simulink model "ACDCMG_woPV"  (R2022a)
settings: Solver=FixedStepAuto  StartTime=0.0  StopTime=0.2  FixedStep=Ts  MaxStep=1e-2  RelTol=1e-3
InitFcn:
  | Set_parameters_R2018
values from neighbouring files (symbols this model uses):
  D_invs = 0.05    [Set_parameters_R2018.m]
  dis11 = 3    [Set_parameters_R2018.m]
  dis14 = 2    [Set_parameters_R2018.m]
  dis2 = 0.2    [Set_parameters_R2018.m]
  dis3 = 0.15    [Set_parameters_R2018.m]
  dis4 = 0.4    [Set_parameters_R2018.m]
  dis5 = 0.4    [Set_parameters_R2018.m]
  dis6 = 0.4    [Set_parameters_R2018.m]
  dis8 = 2    [Set_parameters_R2018.m]
  Fnom = 60    [Set_parameters_R2018.m]
  H_invs = 6    [Set_parameters_R2018.m]
  max_min = 1    [Set_parameters_R2018.m]
  P_Load_3 = S_Load_3* PF_Load_3    (= 25500)    [Set_parameters_R2018.m]
  P_nom_inv = 3e3    (= 3000)    [Set_parameters_R2018.m]
  Pnom_T1 = 1.5e6    (= 1500000)    [Set_parameters_R2018.m]
  Pnom_T2 = 1.5e6    (= 1500000)    [Set_parameters_R2018.m]
  Pnom_T3 = 4e6    (= 4000000)    [Set_parameters_R2018.m]
  Ql_Load_3 = S_Load_3 * sin(acos(PF_Load_3))    [Set_parameters_R2018.m]
  R_Load_9 = (Vnom_prim * 1.35)^2 / P_Load_9    (= 1084.6153125)    [Set_parameters_R2018.m]
  R_Load_DC = Vnom_DC^2/ P_Load_DC    (= 45)    [Set_parameters_R2018.m]
  Rl = 0.394    [Set_parameters_R2018.m]
  Rls = 0.198    [Set_parameters_R2018.m]
  Ts = Ts_Power    (= 6.94444444444e-06)    [Set_parameters_R2018.m]
  Ts_Control = 6*Ts_Power    (= 4.16666666667e-05)    [Set_parameters_R2018.m]
  Ts_Power = 1/(24*Fnom)/100    (= 6.94444444444e-06)    [Set_parameters_R2018.m]
  V1_LL_T3 = 69e3    (= 69000)    [Set_parameters_R2018.m]
  Vnom_DC = 300    [Set_parameters_R2018.m]
  Vnom_Diesel = 2.4e3    (= 2400)    [Set_parameters_R2018.m]
  Vnom_prim = 13.8e3    (= 13800)    [Set_parameters_R2018.m]
  Vnom_sec = 220    [Set_parameters_R2018.m]
  Vnom_ter_AC_DC = 150    [Set_parameters_R2018.m]
  Xl = 0.1168    [Set_parameters_R2018.m]
  Xls = 0.1089    [Set_parameters_R2018.m]
undefined symbols (not defined in the file or in its folder): D1, Delta, DiscIntNeverNeededParam, ee_sli_rtmsupport, fn, gcbh, Ion, Lithium, S, sigbuilder_block, VnInv
libraries: powerlib_extras x55, spsCurrentMeasurementLib x53, powerlib_meascontrol x42, spsSeriesRLCBranchLib x32, spsVoltageMeasurementLib x31, spsRMSLib x29, spsThreePhaseVIMeasurementLib x24, simulink x21, spsThreePhaseSeriesRLCBranchLib x19, spsPower3phInstantaneousLib x15, spsPowerLib x12, spsGroundLib x11
(part 9 of 9)

== system ACDCMG_woPV/Grid Bi-directional Converter 1.2 300 (DC) // 150 V (AC) P_nom 3kW3/Control of Inverter/V//F/Subsystem ==
  note: w
  e : Inport
  io : Inport  Port=2
  i : Inport  Port=3
  fcmd : Inport  Port=4
  Constant1 : Constant  Value=2*pi
  Demux : Demux  Outputs=3
  Demux1 : Demux  Outputs=3
  Demux2 : Demux  Outputs=3
  Discrete Virtual PLL : powerlib_extras/Discrete  Control Blocks/Discrete Virtual PLL  Commented=on  Freq=50  Phase=0  Ts=Ts_Control
      settings: SourceProductBaseCode=PS
  Gain1 : Gain  Gain=2*pi
  Integrator : Integrator
  Math Function : Math  Operator=mod  SignedPower=on
  Scope : Scope
  Scope3 : Scope
  Terminator1 : Terminator
  Terminator2 : Terminator
  Terminator3 : Terminator
  Terminator4 : Terminator  Commented=on
  abc to dq0 : powerlib_meascontrol/Transformations/abc to dq0  Alignment=90 degrees behind phase A axis
  abc to dq1 : powerlib_meascontrol/Transformations/abc to dq0  Alignment=90 degrees behind phase A axis
  abc to dq2 : powerlib_meascontrol/Transformations/abc to dq0  Alignment=90 degrees behind phase A axis
  abc_to_dq0 Transformation2 : powerlib_extras/Measurements/abc_to_dq0 Transformation  Commented=on
      settings: SourceProductBaseCode=PS
  pack6 Scope1 : Scope  NumInputPorts=2
  ed : Outport
  eq : Outport  Port=2
  iod : Outport  Port=3
  ioq : Outport  Port=4
  id : Outport  Port=5
  iq : Outport  Port=6
  w : Outport  Port=7
  "wt " : Outport  Port=8
  wires:
  e/1 -> abc to dq0/1
  i/1 -> abc to dq1/1
  fcmd/1 -> Gain1/1
  Math Function/1 -> Scope3/1, abc to dq1/2, abc to dq2/2, abc to dq0/2, "wt "/1
  abc to dq0/1 -> Demux/1
  Demux1/1 -> id/1
  Demux1/2 -> iq/1
  Demux1/3 -> Terminator3/1
  Demux/1 -> ed/1
  Demux/2 -> eq/1
  Demux/3 -> Terminator1/1
  abc to dq1/1 -> Demux1/1
  Constant1/1 -> Math Function/2
  Integrator/1 -> Math Function/1
  io/1 -> abc to dq2/1
  abc to dq2/1 -> Demux2/1
  Demux2/3 -> Terminator2/1
  Gain1/1 -> Scope/1, w/1, Integrator/1
  Discrete Virtual PLL/2 -> Terminator4/1
  Demux2/1 -> pack6 Scope1/1, iod/1
  Demux2/2 -> pack6 Scope1/2, ioq/1

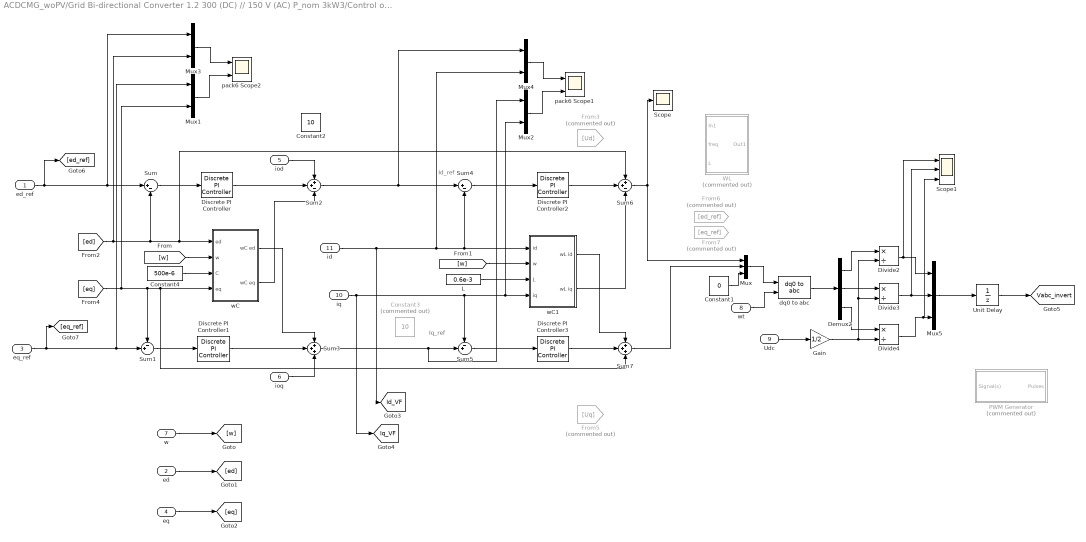
== system ACDCMG_woPV/Grid Bi-directional Converter 1.2 300 (DC) // 150 V (AC) P_nom 3kW3/Control of Inverter/V//F/UIcontrol ==
  note: Id_ref
  note: Iq_ref
  ed_ref : Inport
  ed : Inport  Port=2
  eq_ref : Inport  Port=3
  eq : Inport  Port=4
  iod : Inport  Port=5
  ioq : Inport  Port=6
  w : Inport  Port=7
  "wt " : Inport  Port=8
  Udc : Inport  Port=9
  iq : Inport  Port=10
  id : Inport  Port=11
  Constant1 : Constant  Value=0
  Constant2 : Constant  Value=10
  Constant3 : Constant  Commented=on  Value=10
  Constant4 : Constant  Value=500e-6
  Demux2 : Demux  Outputs=3
  Discrete PI Controller : powerlib_extras/Discrete  Control Blocks/Discrete PI Controller  Kp=5  Ki=50  Par_Limits=[1e6 -1e6]  Init=0  Ts=Ts_Control
  Discrete PI Controller1 : powerlib_extras/Discrete  Control Blocks/Discrete PI Controller  Kp=5  Ki=50  Par_Limits=[1e6 -1e6]  Init=0  Ts=Ts_Control
  Discrete PI Controller2 : powerlib_extras/Discrete  Control Blocks/Discrete PI Controller  Kp=25  Ki=1800  Par_Limits=[1e6 -1e6]  Init=0  Ts=Ts_Control
  Discrete PI Controller3 : powerlib_extras/Discrete  Control Blocks/Discrete PI Controller  Kp=25  Ki=1800  Par_Limits=[1e6 -1e6]  Init=0  Ts=Ts_Control
  Divide2 : Product  Inputs=*/
  Divide3 : Product  Inputs=*/
  Divide4 : Product  Inputs=*/
  From3 : From  Commented=on  GotoTag=Ud
  From5 : From  Commented=on  GotoTag=Uq
  From6 : From  Commented=on  GotoTag=ed_ref
  From7 : From  Commented=on  GotoTag=eq_ref
  Gain : Gain  Gain=1/2
  L : Constant  Value=0.6e-3
  Mux : Mux  Inputs=3
  Mux{1..4} (4 alike) : Mux  Inputs=2
  Mux5 : Mux  Inputs=3
  PWM Generator : Subsystem  Commented=on  AncestorBlock="powerlib_extras/Control  Blocks/PWM Generator"  DialogController=POWERSYS.PowerSysDialog  mask(PWM Generator){GeneratorMode=3-arm  bridge (6 pulses), Fc=10000, Internal=off, mIndex=0.4, Freq=50, Phase=0}
      mask prompts: GeneratorMode "Generator Mode"; Fc "Carrier frequency (Hz):"; Internal "Internal generation of modulating signal(s)"; mIndex "Modulation index  (0<m<1) :"; Freq "Frequency of output voltage (Hz)"; Phase "Phase of output voltage (degrees)"
      mask help:
      | This block generates pulses for carrier-based PWM (Pulse Width Modulation), self-commutated IGBTs,GTOs or FETs bridges.
      |
      | Depending on the number of bridge arms selected in the "Generator Mode" parameter, the block can be used either for single-phase or three-phase PWM control.
      mask init: same as ACDCMG_woPV/Grid Bi-directional Converter 1.2 300 (DC) // 150 V (AC) P_nom 3kW/Control of Inverter/V//F/UIcontrol/PWM Generator
      mask Help: web(psbhelp)
      mask TypeOptions GeneratorMode: 1-arm  bridge (2 pulses) | 2-arm  bridge (4 pulses) | 3-arm  bridge (6 pulses) | Double 3-arm  bridges (12 pulses)
      mask Callback Internal: p3=get_param(gcb,'Internal');if strcmp(p3,'on');visible={'on','on','on','on','on','on'};else;visible={'on','on','on','off','off','off'};end;set_param(gcb,'MaskVisibilities',visible)
  Scope : Scope
  Scope1 : Scope  NumInputPorts=3
  Sum : Sum  Inputs=|+-
  Sum1 : Sum  Inputs=-+|
  Sum2 : Sum  Inputs=++-
  Sum3 : Sum  Inputs=+++
  Sum4 : Sum  Inputs=|+-
  Sum5 : Sum  Inputs=-+|
  Sum6 : Sum  Inputs=++-
  Sum7 : Sum  Inputs=+++
  Unit Delay : UnitDelay  SampleTime=-1  HasFrameUpgradeWarning=on
  WL : Subsystem  Commented=on
  dq0 to abc : powerlib_meascontrol/Transformations/dq0 to abc  Alignment=90 degrees behind phase A axis
  pack6 Scope1 : Scope  NumInputPorts=2
  pack6 Scope2 : Scope  NumInputPorts=2
  wC : Subsystem
  wC1 : Subsystem
  tag scope: Id_VF=global, Iq_VF=global, Vabc_invert=global
  wires:
  ed_ref/1 -> [ed_ref], Mux3/1, Sum/1
  Sum/1 -> Discrete PI Controller/1
  Mux/1 -> dq0 to abc/1
  "wt "/1 -> dq0 to abc/2
  Mux5/1 -> Unit Delay/1
  Demux2/1 -> Divide2/1
  Demux2/2 -> Divide3/1
  Gain/1 -> Divide3/2, Divide2/2, Divide4/2
  Divide4/1 -> Scope1/3, Mux5/3
  Divide2/1 -> Mux5/1, Scope1/1
  Demux2/3 -> Divide4/1
  Divide3/1 -> Scope1/2, Mux5/2
  dq0 to abc/1 -> Demux2/1
  Udc/1 -> Gain/1
  Constant4/1 -> wC/3(C)
  [w] -> wC/2(w)
  [eq] -> Mux1/2, Sum7/3, wC/4(eq), Sum1/1
  Sum1/1 -> Discrete PI Controller1/1
  eq_ref/1 -> [eq_ref], Mux1/1, Sum1/2
  L/1 -> wC1/3(L)
  Sum5/1 -> Discrete PI Controller3/1
  Sum4/1 -> Discrete PI Controller2/1
  Discrete PI Controller3/1 -> Sum7/2
  Discrete PI Controller2/1 -> Sum6/2
  w/1 -> [w]
  [w] -> wC1/2(w)
  ed/1 -> [ed]
  eq/1 -> [eq]
  Sum6/1 -> Mux/1, Scope/1
  Constant1/1 -> Mux/3
  Mux4/1 -> pack6 Scope1/1
  Mux2/1 -> pack6 Scope1/2
  iq/1 -> [Iq_VF], Sum5/1, wC1/4(iq), Mux2/2
  Discrete PI Controller/1 -> Sum2/2
  Discrete PI Controller1/1 -> Sum3/2
  id/1 -> [Id_VF], Mux4/2, wC1/1(id), Sum4/2
  Mux3/1 -> pack6 Scope2/1
  Mux1/1 -> pack6 Scope2/2
  wC/1(wC ed) -> Sum3/1
  ioq/1 -> Sum3/3
  iod/1 -> Sum2/1
  wC/2(wC eq) -> Sum2/3
  wC1/1(wL id) -> Sum7/1
  wC1/2(wL iq) -> Sum6/3
  [ed] -> Sum6/1, wC/1(ed), Sum/2, Mux3/2
  Sum2/1 -> Mux4/1, Sum4/1
  Sum3/1 -> Mux2/1, Sum5/2
  Unit Delay/1 -> [Vabc_invert]
  Sum7/1 -> Mux/2

== system ACDCMG_woPV/Inverter 300 (DC) // 150 V (AC) P_nom 3kW4/Control of Inverter/Subsystem2/Subsystem1 ==
  note: Iq* = 2/3*( P*Vq - Q*Vd ) / ( Vd^2 + Vq^2 )
  note: Reference computation:
  note: Id* = 2/3* ( P*Vd + Q*Vq ) / ( Vd^2 + Vq^2 )
  P_ref : Inport  PortDimensions=1
  Q_ref : Inport  Port=2  PortDimensions=1
  Vd : Inport  Port=3  PortDimensions=1
  Vq : Inport  Port=4  PortDimensions=1
  Constant1 : Constant  Commented=on  Value=0
  Demux3 : Demux  Outputs=2
      settings: DisplayOption=none
  Fcn3 : Fcn  Expr=u(1)*u(1)+u(2)*u(2)
  Gain : Gain  Gain=2/3
  Mux1 : Mux  Inputs=2
  Mux3 : Mux  Inputs=2
  Product{2..5} (4 alike) : Product  InputSameDT=on  SaturateOnIntegerOverflow=on  OutDataTypeStr=Inherit: Same as first input
  Product6 : Product  Inputs=*/  InputSameDT=on  SaturateOnIntegerOverflow=on  OutDataTypeStr=Inherit: Same as first input
  Scope3 : Scope  NumInputPorts=2
  Sum : Sum  InputSameDT=on  SaturateOnIntegerOverflow=on  OutDataTypeStr=Inherit: Same as first input
  Sum1 : Sum  Inputs=+-  InputSameDT=on  SaturateOnIntegerOverflow=on  OutDataTypeStr=Inherit: Same as first input
  Terminator : Terminator  Commented=on
  Id_ref : Outport
  Iq_ref : Outport  Port=2
  wires:
  Vq/1 -> Mux1/2, Product4/2, Product3/1
  Demux3/1 -> Scope3/1, Id_ref/1
  Mux1/1 -> Fcn3/1
  Product3/1 -> Sum/2
  Mux3/1 -> Gain/1
  Vd/1 -> Mux1/1, Product5/2, Product2/1
  Product4/1 -> Sum1/1
  Product6/1 -> Demux3/1
  Fcn3/1 -> Product6/2
  Demux3/2 -> Scope3/2, Iq_ref/1
  P_ref/1 -> Product2/2, Product4/1
  Gain/1 -> Product6/1
  Product2/1 -> Sum/1
  Q_ref/1 -> Product5/1, Product3/2
  Sum1/1 -> Mux3/2
  Product5/1 -> Sum1/2
  Sum/1 -> Mux3/1

== system ACDCMG_woPV/Inverter 300 (DC) // 150 V (AC) P_nom 3kW4/Control of Inverter/Subsystem2/WL ==
  In1 : Inport
  freq : Inport  Port=2
  L : Inport  Port=3
  2pai : Constant  Value=2*pi
  Product : Product  Inputs=**
  Product1 : Product  Inputs=***
  Out1 : Outport
  wires:
  2pai/1 -> Product/2
  L/1 -> Product1/3
  freq/1 -> Product/1
  Product1/1 -> Out1/1
  Product/1 -> Product1/2
  In1/1 -> Product1/1

== system ACDCMG_woPV/Inverter 300 (DC) // 150 V (AC) P_nom 3kW4/Control of Inverter/Subsystem2/WL1 ==
  In1 : Inport
  freq : Inport  Port=2
  L : Inport  Port=3
  2pai : Constant  Value=2*pi
  Product : Product
  Product1 : Product  Inputs=3
  Out1 : Outport
  wires:
  2pai/1 -> Product/2
  L/1 -> Product1/3
  freq/1 -> Product/1
  Product1/1 -> Out1/1
  Product/1 -> Product1/2
  In1/1 -> Product1/1

== system ACDCMG_woPV/Inverter 300 (DC) // 150 V (AC) P_nom 3kW4/Control of Inverter/V//F/Subsystem ==
  note: w
  e : Inport
  io : Inport  Port=2
  i : Inport  Port=3
  fcmd : Inport  Port=4
  Constant1 : Constant  Value=2*pi
  Demux : Demux  Outputs=3
  Demux1 : Demux  Outputs=3
  Demux2 : Demux  Outputs=3
  Discrete Virtual PLL : powerlib_extras/Discrete  Control Blocks/Discrete Virtual PLL  Commented=on  Freq=50  Phase=0  Ts=Ts_Control
      settings: SourceProductBaseCode=PS
  Gain1 : Gain  Gain=2*pi
  Integrator : Integrator
  Math Function : Math  Operator=mod  SignedPower=on
  Scope : Scope
  Scope3 : Scope
  Terminator1 : Terminator
  Terminator2 : Terminator
  Terminator3 : Terminator
  Terminator4 : Terminator  Commented=on
  abc to dq0 : powerlib_meascontrol/Transformations/abc to dq0  Alignment=90 degrees behind phase A axis
  abc to dq1 : powerlib_meascontrol/Transformations/abc to dq0  Alignment=90 degrees behind phase A axis
  abc to dq2 : powerlib_meascontrol/Transformations/abc to dq0  Alignment=90 degrees behind phase A axis
  abc_to_dq0 Transformation2 : powerlib_extras/Measurements/abc_to_dq0 Transformation  Commented=on
      settings: SourceProductBaseCode=PS
  pack6 Scope1 : Scope  NumInputPorts=2
  ed : Outport
  eq : Outport  Port=2
  iod : Outport  Port=3
  ioq : Outport  Port=4
  id : Outport  Port=5
  iq : Outport  Port=6
  w : Outport  Port=7
  "wt " : Outport  Port=8
  wires:
  e/1 -> abc to dq0/1
  i/1 -> abc to dq1/1
  fcmd/1 -> Gain1/1
  Math Function/1 -> Scope3/1, abc to dq1/2, abc to dq2/2, abc to dq0/2, "wt "/1
  abc to dq0/1 -> Demux/1
  Demux1/1 -> id/1
  Demux1/2 -> iq/1
  Demux1/3 -> Terminator3/1
  Demux/1 -> ed/1
  Demux/2 -> eq/1
  Demux/3 -> Terminator1/1
  abc to dq1/1 -> Demux1/1
  Constant1/1 -> Math Function/2
  Integrator/1 -> Math Function/1
  io/1 -> abc to dq2/1
  abc to dq2/1 -> Demux2/1
  Demux2/3 -> Terminator2/1
  Gain1/1 -> Scope/1, w/1, Integrator/1
  Discrete Virtual PLL/2 -> Terminator4/1
  Demux2/1 -> pack6 Scope1/1, iod/1
  Demux2/2 -> pack6 Scope1/2, ioq/1

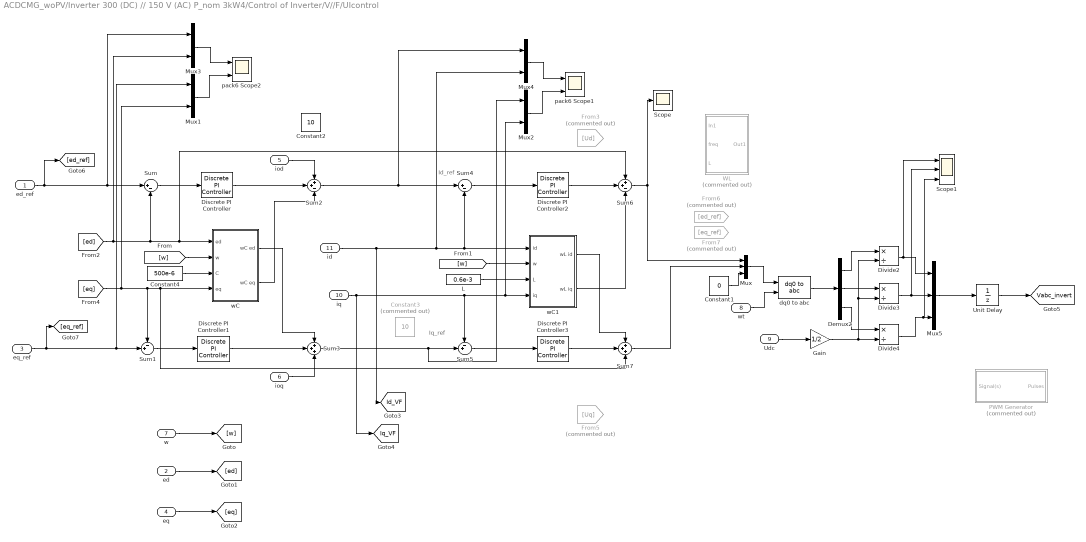
== system ACDCMG_woPV/Inverter 300 (DC) // 150 V (AC) P_nom 3kW4/Control of Inverter/V//F/UIcontrol ==
  note: Id_ref
  note: Iq_ref
  ed_ref : Inport
  ed : Inport  Port=2
  eq_ref : Inport  Port=3
  eq : Inport  Port=4
  iod : Inport  Port=5
  ioq : Inport  Port=6
  w : Inport  Port=7
  "wt " : Inport  Port=8
  Udc : Inport  Port=9
  iq : Inport  Port=10
  id : Inport  Port=11
  Constant1 : Constant  Value=0
  Constant2 : Constant  Value=10
  Constant3 : Constant  Commented=on  Value=10
  Constant4 : Constant  Value=500e-6
  Demux2 : Demux  Outputs=3
  Discrete PI Controller : powerlib_extras/Discrete  Control Blocks/Discrete PI Controller  Kp=5  Ki=50  Par_Limits=[1e6 -1e6]  Init=0  Ts=Ts_Control
  Discrete PI Controller1 : powerlib_extras/Discrete  Control Blocks/Discrete PI Controller  Kp=5  Ki=50  Par_Limits=[1e6 -1e6]  Init=0  Ts=Ts_Control
  Discrete PI Controller2 : powerlib_extras/Discrete  Control Blocks/Discrete PI Controller  Kp=25  Ki=1800  Par_Limits=[1e6 -1e6]  Init=0  Ts=Ts_Control
  Discrete PI Controller3 : powerlib_extras/Discrete  Control Blocks/Discrete PI Controller  Kp=25  Ki=1800  Par_Limits=[1e6 -1e6]  Init=0  Ts=Ts_Control
  Divide2 : Product  Inputs=*/
  Divide3 : Product  Inputs=*/
  Divide4 : Product  Inputs=*/
  From3 : From  Commented=on  GotoTag=Ud
  From5 : From  Commented=on  GotoTag=Uq
  From6 : From  Commented=on  GotoTag=ed_ref
  From7 : From  Commented=on  GotoTag=eq_ref
  Gain : Gain  Gain=1/2
  L : Constant  Value=0.6e-3
  Mux : Mux  Inputs=3
  Mux{1..4} (4 alike) : Mux  Inputs=2
  Mux5 : Mux  Inputs=3
  PWM Generator : Subsystem  Commented=on  AncestorBlock="powerlib_extras/Control  Blocks/PWM Generator"  DialogController=POWERSYS.PowerSysDialog  mask(PWM Generator){GeneratorMode=3-arm  bridge (6 pulses), Fc=10000, Internal=off, mIndex=0.4, Freq=50, Phase=0}
      mask prompts: GeneratorMode "Generator Mode"; Fc "Carrier frequency (Hz):"; Internal "Internal generation of modulating signal(s)"; mIndex "Modulation index  (0<m<1) :"; Freq "Frequency of output voltage (Hz)"; Phase "Phase of output voltage (degrees)"
      mask help:
      | This block generates pulses for carrier-based PWM (Pulse Width Modulation), self-commutated IGBTs,GTOs or FETs bridges.
      |
      | Depending on the number of bridge arms selected in the "Generator Mode" parameter, the block can be used either for single-phase or three-phase PWM control.
      mask init: same as ACDCMG_woPV/Grid Bi-directional Converter 1.2 300 (DC) // 150 V (AC) P_nom 3kW/Control of Inverter/V//F/UIcontrol/PWM Generator
      mask Help: web(psbhelp)
      mask TypeOptions GeneratorMode: 1-arm  bridge (2 pulses) | 2-arm  bridge (4 pulses) | 3-arm  bridge (6 pulses) | Double 3-arm  bridges (12 pulses)
      mask Callback Internal: p3=get_param(gcb,'Internal');if strcmp(p3,'on');visible={'on','on','on','on','on','on'};else;visible={'on','on','on','off','off','off'};end;set_param(gcb,'MaskVisibilities',visible)
  Scope : Scope
  Scope1 : Scope  NumInputPorts=3
  Sum : Sum  Inputs=|+-
  Sum1 : Sum  Inputs=-+|
  Sum2 : Sum  Inputs=++-
  Sum3 : Sum  Inputs=+++
  Sum4 : Sum  Inputs=|+-
  Sum5 : Sum  Inputs=-+|
  Sum6 : Sum  Inputs=++-
  Sum7 : Sum  Inputs=+++
  Unit Delay : UnitDelay  SampleTime=-1  HasFrameUpgradeWarning=on
  WL : Subsystem  Commented=on
  dq0 to abc : powerlib_meascontrol/Transformations/dq0 to abc  Alignment=90 degrees behind phase A axis
  pack6 Scope1 : Scope  NumInputPorts=2
  pack6 Scope2 : Scope  NumInputPorts=2
  wC : Subsystem
  wC1 : Subsystem
  tag scope: Id_VF=global, Iq_VF=global, Vabc_invert=global
  wires:
  ed_ref/1 -> [ed_ref], Mux3/1, Sum/1
  Sum/1 -> Discrete PI Controller/1
  Mux/1 -> dq0 to abc/1
  "wt "/1 -> dq0 to abc/2
  Mux5/1 -> Unit Delay/1
  Demux2/1 -> Divide2/1
  Demux2/2 -> Divide3/1
  Gain/1 -> Divide3/2, Divide2/2, Divide4/2
  Divide4/1 -> Scope1/3, Mux5/3
  Divide2/1 -> Mux5/1, Scope1/1
  Demux2/3 -> Divide4/1
  Divide3/1 -> Scope1/2, Mux5/2
  dq0 to abc/1 -> Demux2/1
  Udc/1 -> Gain/1
  Constant4/1 -> wC/3(C)
  [w] -> wC/2(w)
  [eq] -> Mux1/2, Sum7/3, wC/4(eq), Sum1/1
  Sum1/1 -> Discrete PI Controller1/1
  eq_ref/1 -> [eq_ref], Mux1/1, Sum1/2
  L/1 -> wC1/3(L)
  Sum5/1 -> Discrete PI Controller3/1
  Sum4/1 -> Discrete PI Controller2/1
  Discrete PI Controller3/1 -> Sum7/2
  Discrete PI Controller2/1 -> Sum6/2
  w/1 -> [w]
  [w] -> wC1/2(w)
  ed/1 -> [ed]
  eq/1 -> [eq]
  Sum6/1 -> Mux/1, Scope/1
  Constant1/1 -> Mux/3
  Mux4/1 -> pack6 Scope1/1
  Mux2/1 -> pack6 Scope1/2
  iq/1 -> [Iq_VF], Sum5/1, wC1/4(iq), Mux2/2
  Discrete PI Controller/1 -> Sum2/2
  Discrete PI Controller1/1 -> Sum3/2
  id/1 -> [Id_VF], Mux4/2, wC1/1(id), Sum4/2
  Mux3/1 -> pack6 Scope2/1
  Mux1/1 -> pack6 Scope2/2
  wC/1(wC ed) -> Sum3/1
  ioq/1 -> Sum3/3
  iod/1 -> Sum2/1
  wC/2(wC eq) -> Sum2/3
  wC1/1(wL id) -> Sum7/1
  wC1/2(wL iq) -> Sum6/3
  [ed] -> Sum6/1, wC/1(ed), Sum/2, Mux3/2
  Sum2/1 -> Mux4/1, Sum4/1
  Sum3/1 -> Mux2/1, Sum5/2
  Unit Delay/1 -> [Vabc_invert]
  Sum7/1 -> Mux/2

== system ACDCMG_woPV/Grid Bi-directional Converter 1.2 300 (DC) // 150 V (AC) P_nom 3kW/Control of Inverter/V//F/UIcontrol/PWM Generator ==
  note: PWM Generator
  note: Pierre Giroux, Gilbert Sybille
      | Power System Laboratory, IREQ
      | Hydro-Quebec
  Signal(s) : Inport  PortDimensions=Signal_PortWidth
  BL4 : Logic  Operator=NOT  Inputs=1
  BL5 : Logic  Operator=NOT  Inputs=1
  Constant : Constant  Value=Internal_Phase
  Constant1 : Constant  Value=Internal
  Data Type Conversion : DataTypeConversion  OutDataTypeStr=double
  Data Type Conversion1 : DataTypeConversion  OutDataTypeStr=boolean
  Data Type Conversion2 : DataTypeConversion  OutDataTypeStr=boolean
  Gain : Gain  Gain=2*pi*Freq  SaturateOnIntegerOverflow=on  OutDataTypeStr=Inherit: Same as input  ParamDataTypeStr=Inherit: Same as input
  Gain2 : Gain  Gain=pi/180  SaturateOnIntegerOverflow=on  OutDataTypeStr=Inherit: Same as input  ParamDataTypeStr=Inherit: Same as input
  Gain3 : Gain  Gain=-1  SaturateOnIntegerOverflow=on  OutDataTypeStr=Inherit: Same as input  ParamDataTypeStr=Inherit: Same as input
  Mux : Mux  Inputs=2
  Mux1 : Mux  Inputs=2
  Mux2 : Mux  Inputs=2
  Product : Product  InputSameDT=on  SaturateOnIntegerOverflow=on  OutDataTypeStr=Inherit: Same as first input
  Relational Operator : RelationalOperator  ZeroCross=off
  Relational Operator1 : RelationalOperator  ZeroCross=off
  Select1A : Selector  InputPortWidth=Select1_PortWidth  IndexOptions=Index vector (dialog)  Indices=Select1_Elements  OutputSizes=1
  Select1B : Selector  InputPortWidth=Select1_PortWidth  IndexOptions=Index vector (dialog)  Indices=Select1_Elements  OutputSizes=1
  Select3 : Selector  InputPortWidth=Select3_PortWidth  IndexOptions=Index vector (dialog)  Indices=Select3_Elements  OutputSizes=1
  Sum : Sum  Inputs=+++  InputSameDT=on  SaturateOnIntegerOverflow=on  OutDataTypeStr=Inherit: Same as first input
  Switch : Switch  Threshold=0.5  SaturateOnIntegerOverflow=off
  Triangle : simulink/Sources/Repeating Sequence  rep_seq_t=[0 1/Fc/4 3/Fc/4 1/Fc]  rep_seq_y=[0 -1 1 0]
  Trigonometric Function : Trigonometry
  m3 : Constant  Value=Phase
  m4 : Constant  Value=mIndex
  t : Clock
  Pulses : Outport
  wires:
  Data Type Conversion2/1 -> Mux1/1, BL5/1
  Relational Operator1/1 -> Data Type Conversion2/1
  Data Type Conversion1/1 -> Mux/1, BL4/1
  Relational Operator/1 -> Data Type Conversion1/1
  Data Type Conversion/1 -> Pulses/1
  Select3/1 -> Data Type Conversion/1
  t/1 -> Gain/1
  Gain/1 -> Sum/1
  Gain2/1 -> Sum/2
  m3/1 -> Gain2/1
  Constant/1 -> Sum/3
  m4/1 -> Product/1
  Sum/1 -> Trigonometric Function/1
  Trigonometric Function/1 -> Product/2
  Signal(s)/1 -> Switch/3
  Constant1/1 -> Switch/2
  Product/1 -> Switch/1
  Gain3/1 -> Relational Operator1/1
  BL4/1 -> Mux/2
  BL5/1 -> Mux1/2
  Mux/1 -> Select1A/1
  Mux1/1 -> Select1B/1
  Select1A/1 -> Mux2/1
  Select1B/1 -> Mux2/2
  Mux2/1 -> Select3/1
  Switch/1 -> Gain3/1, Relational Operator/1
  Triangle/1 -> Relational Operator1/2, Relational Operator/2

== system ACDCMG_woPV/Grid Bi-directional Converter 1.2 300 (DC) // 150 V (AC) P_nom 3kW/Control of Inverter/V//F/UIcontrol/WL ==
  In1 : Inport
  freq : Inport  Port=2
  L : Inport  Port=3
  2pai : Constant  Value=2*pi
  Product : Product  Inputs=**
  Product1 : Product  Inputs=***
  Out1 : Outport
  wires:
  2pai/1 -> Product/2
  L/1 -> Product1/3
  freq/1 -> Product/1
  Product1/1 -> Out1/1
  Product/1 -> Product1/2
  In1/1 -> Product1/1

== system ACDCMG_woPV/Grid Bi-directional Converter 1.2 300 (DC) // 150 V (AC) P_nom 3kW/Control of Inverter/V//F/UIcontrol/wC ==
  ed : Inport
  w : Inport  Port=2
  C : Inport  Port=3
  eq : Inport  Port=4
  Product1 : Product  Inputs=3
  Product2 : Product  Inputs=3
  wC ed : Outport
  wC eq : Outport  Port=2
  wires:
  C/1 -> Product1/3, Product2/2
  Product1/1 -> wC ed/1
  w/1 -> Product1/2, Product2/1
  ed/1 -> Product1/1
  eq/1 -> Product2/3
  Product2/1 -> wC eq/1

== system ACDCMG_woPV/Grid Bi-directional Converter 1.2 300 (DC) // 150 V (AC) P_nom 3kW/Control of Inverter/V//F/UIcontrol/wC1 ==
  id : Inport
  w : Inport  Port=2
  L : Inport  Port=3
  iq : Inport  Port=4
  Product1 : Product  Inputs=***
  Product2 : Product  Inputs=***
  wL id : Outport
  wL iq : Outport  Port=2
  wires:
  L/1 -> Product1/3, Product2/2
  Product1/1 -> wL id/1
  w/1 -> Product1/2, Product2/1
  id/1 -> Product1/1
  iq/1 -> Product2/3
  Product2/1 -> wL iq/1

== system ACDCMG_woPV/Grid Bi-directional Converter 1.2 300 (DC) // 150 V (AC) P_nom 3kW1/Control of Inverter/V//F/UIcontrol/PWM Generator ==
  note: PWM Generator
  note: Pierre Giroux, Gilbert Sybille
      | Power System Laboratory, IREQ
      | Hydro-Quebec
  Signal(s) : Inport  PortDimensions=Signal_PortWidth
  BL4 : Logic  Operator=NOT  Inputs=1
  BL5 : Logic  Operator=NOT  Inputs=1
  Constant : Constant  Value=Internal_Phase
  Constant1 : Constant  Value=Internal
  Data Type Conversion : DataTypeConversion  OutDataTypeStr=double
  Data Type Conversion1 : DataTypeConversion  OutDataTypeStr=boolean
  Data Type Conversion2 : DataTypeConversion  OutDataTypeStr=boolean
  Gain : Gain  Gain=2*pi*Freq  SaturateOnIntegerOverflow=on  OutDataTypeStr=Inherit: Same as input  ParamDataTypeStr=Inherit: Same as input
  Gain2 : Gain  Gain=pi/180  SaturateOnIntegerOverflow=on  OutDataTypeStr=Inherit: Same as input  ParamDataTypeStr=Inherit: Same as input
  Gain3 : Gain  Gain=-1  SaturateOnIntegerOverflow=on  OutDataTypeStr=Inherit: Same as input  ParamDataTypeStr=Inherit: Same as input
  Mux : Mux  Inputs=2
  Mux1 : Mux  Inputs=2
  Mux2 : Mux  Inputs=2
  Product : Product  InputSameDT=on  SaturateOnIntegerOverflow=on  OutDataTypeStr=Inherit: Same as first input
  Relational Operator : RelationalOperator  ZeroCross=off
  Relational Operator1 : RelationalOperator  ZeroCross=off
  Select1A : Selector  InputPortWidth=Select1_PortWidth  IndexOptions=Index vector (dialog)  Indices=Select1_Elements  OutputSizes=1
  Select1B : Selector  InputPortWidth=Select1_PortWidth  IndexOptions=Index vector (dialog)  Indices=Select1_Elements  OutputSizes=1
  Select3 : Selector  InputPortWidth=Select3_PortWidth  IndexOptions=Index vector (dialog)  Indices=Select3_Elements  OutputSizes=1
  Sum : Sum  Inputs=+++  InputSameDT=on  SaturateOnIntegerOverflow=on  OutDataTypeStr=Inherit: Same as first input
  Switch : Switch  Threshold=0.5  SaturateOnIntegerOverflow=off
  Triangle : simulink/Sources/Repeating Sequence  rep_seq_t=[0 1/Fc/4 3/Fc/4 1/Fc]  rep_seq_y=[0 -1 1 0]
  Trigonometric Function : Trigonometry
  m3 : Constant  Value=Phase
  m4 : Constant  Value=mIndex
  t : Clock
  Pulses : Outport
  wires:
  Data Type Conversion2/1 -> Mux1/1, BL5/1
  Relational Operator1/1 -> Data Type Conversion2/1
  Data Type Conversion1/1 -> Mux/1, BL4/1
  Relational Operator/1 -> Data Type Conversion1/1
  Data Type Conversion/1 -> Pulses/1
  Select3/1 -> Data Type Conversion/1
  t/1 -> Gain/1
  Gain/1 -> Sum/1
  Gain2/1 -> Sum/2
  m3/1 -> Gain2/1
  Constant/1 -> Sum/3
  m4/1 -> Product/1
  Sum/1 -> Trigonometric Function/1
  Trigonometric Function/1 -> Product/2
  Signal(s)/1 -> Switch/3
  Constant1/1 -> Switch/2
  Product/1 -> Switch/1
  Gain3/1 -> Relational Operator1/1
  BL4/1 -> Mux/2
  BL5/1 -> Mux1/2
  Mux/1 -> Select1A/1
  Mux1/1 -> Select1B/1
  Select1A/1 -> Mux2/1
  Select1B/1 -> Mux2/2
  Mux2/1 -> Select3/1
  Switch/1 -> Gain3/1, Relational Operator/1
  Triangle/1 -> Relational Operator1/2, Relational Operator/2

== system ACDCMG_woPV/Grid Bi-directional Converter 1.2 300 (DC) // 150 V (AC) P_nom 3kW1/Control of Inverter/V//F/UIcontrol/WL ==
  In1 : Inport
  freq : Inport  Port=2
  L : Inport  Port=3
  2pai : Constant  Value=2*pi
  Product : Product  Inputs=**
  Product1 : Product  Inputs=***
  Out1 : Outport
  wires:
  2pai/1 -> Product/2
  L/1 -> Product1/3
  freq/1 -> Product/1
  Product1/1 -> Out1/1
  Product/1 -> Product1/2
  In1/1 -> Product1/1

== system ACDCMG_woPV/Grid Bi-directional Converter 1.2 300 (DC) // 150 V (AC) P_nom 3kW1/Control of Inverter/V//F/UIcontrol/wC ==
  ed : Inport
  w : Inport  Port=2
  C : Inport  Port=3
  eq : Inport  Port=4
  Product1 : Product  Inputs=3
  Product2 : Product  Inputs=3
  wC ed : Outport
  wC eq : Outport  Port=2
  wires:
  C/1 -> Product1/3, Product2/2
  Product1/1 -> wC ed/1
  w/1 -> Product1/2, Product2/1
  ed/1 -> Product1/1
  eq/1 -> Product2/3
  Product2/1 -> wC eq/1

== system ACDCMG_woPV/Grid Bi-directional Converter 1.2 300 (DC) // 150 V (AC) P_nom 3kW1/Control of Inverter/V//F/UIcontrol/wC1 ==
  id : Inport
  w : Inport  Port=2
  L : Inport  Port=3
  iq : Inport  Port=4
  Product1 : Product  Inputs=***
  Product2 : Product  Inputs=***
  wL id : Outport
  wL iq : Outport  Port=2
  wires:
  L/1 -> Product1/3, Product2/2
  Product1/1 -> wL id/1
  w/1 -> Product1/2, Product2/1
  id/1 -> Product1/1
  iq/1 -> Product2/3
  Product2/1 -> wL iq/1

== system ACDCMG_woPV/Grid Bi-directional Converter 1.2 300 (DC) // 150 V (AC) P_nom 3kW1/Power Measurement (Three-Phase)/Discrete/Phase-A I/Corrected discrete transport delay ==
  In : Inport
  Add1 : Sum
  Add2 : Sum
  Add3 : Sum
  Delay : Delay  DelayLength=ceil(1/F/Ts)-1
  Gain : Gain  Gain=0.5
  Subtract{1..4} (4 alike) : Sum  Inputs=+-
  Unit Delay1 : UnitDelay  SampleTime=Ts  HasFrameUpgradeWarning=on
  Unit Delay2 : UnitDelay  SampleTime=Ts  HasFrameUpgradeWarning=on
  delta : Gain  Gain=(1/F/Ts) - (ceil(1/F/Ts)-1)
  delta' : Gain  Gain=ceil(1/F/Ts) - (1/F/Ts)
  Out : Outport  VectorParamsAs1DForOutWhenUnconnected=off
  wires:
  Gain/1 -> Out/1
  Add3/1 -> Gain/1
  Add1/1 -> Subtract3/1
  Unit Delay2/1 -> Subtract2/2, Add2/2, Subtract3/2
  delta/1 -> Add1/1
  delta'/1 -> Add2/1
  Subtract2/1 -> delta'/1
  Subtract4/1 -> Add3/2
  In/1 -> Subtract1/1, Unit Delay1/1, Subtract4/1, Delay/1
  Unit Delay1/1 -> Add1/2, Subtract1/2
  Delay/1 -> Unit Delay2/1, Subtract2/1
  Subtract3/1 -> Add3/1
  Subtract1/1 -> delta/1
  Add2/1 -> Subtract4/2

== system ACDCMG_woPV/Grid Bi-directional Converter 1.2 300 (DC) // 150 V (AC) P_nom 3kW1/Power Measurement (Three-Phase)/Discrete/Phase-A V/Corrected discrete transport delay ==
  In : Inport
  Add1 : Sum
  Add2 : Sum
  Add3 : Sum
  Delay : Delay  DelayLength=ceil(1/F/Ts)-1
  Gain : Gain  Gain=0.5
  Subtract{1..4} (4 alike) : Sum  Inputs=+-
  Unit Delay1 : UnitDelay  SampleTime=Ts  HasFrameUpgradeWarning=on
  Unit Delay2 : UnitDelay  SampleTime=Ts  HasFrameUpgradeWarning=on
  delta : Gain  Gain=(1/F/Ts) - (ceil(1/F/Ts)-1)
  delta' : Gain  Gain=ceil(1/F/Ts) - (1/F/Ts)
  Out : Outport  VectorParamsAs1DForOutWhenUnconnected=off
  wires:
  Add2/1 -> Subtract4/2
  Subtract1/1 -> delta/1
  Subtract3/1 -> Add3/1
  Delay/1 -> Subtract2/1, Unit Delay2/1
  Unit Delay1/1 -> Subtract1/2, Add1/2
  In/1 -> Delay/1, Subtract4/1, Unit Delay1/1, Subtract1/1
  Subtract4/1 -> Add3/2
  Subtract2/1 -> delta'/1
  delta'/1 -> Add2/1
  delta/1 -> Add1/1
  Unit Delay2/1 -> Subtract3/2, Add2/2, Subtract2/2
  Add1/1 -> Subtract3/1
  Add3/1 -> Gain/1
  Gain/1 -> Out/1

== system ACDCMG_woPV/Grid Bi-directional Converter 1.2 300 (DC) // 150 V (AC) P_nom 3kW1/Power Measurement (Three-Phase)/Discrete/Phase-B I/Corrected discrete transport delay ==
  In : Inport
  Add1 : Sum
  Add2 : Sum
  Add3 : Sum
  Delay : Delay  DelayLength=ceil(1/F/Ts)-1
  Gain : Gain  Gain=0.5
  Subtract{1..4} (4 alike) : Sum  Inputs=+-
  Unit Delay1 : UnitDelay  SampleTime=Ts  HasFrameUpgradeWarning=on
  Unit Delay2 : UnitDelay  SampleTime=Ts  HasFrameUpgradeWarning=on
  delta : Gain  Gain=(1/F/Ts) - (ceil(1/F/Ts)-1)
  delta' : Gain  Gain=ceil(1/F/Ts) - (1/F/Ts)
  Out : Outport  VectorParamsAs1DForOutWhenUnconnected=off
  wires:
  Add2/1 -> Subtract4/2
  Subtract1/1 -> delta/1
  Subtract3/1 -> Add3/1
  Delay/1 -> Subtract2/1, Unit Delay2/1
  Unit Delay1/1 -> Subtract1/2, Add1/2
  In/1 -> Delay/1, Subtract4/1, Unit Delay1/1, Subtract1/1
  Subtract4/1 -> Add3/2
  Subtract2/1 -> delta'/1
  delta'/1 -> Add2/1
  delta/1 -> Add1/1
  Unit Delay2/1 -> Subtract3/2, Add2/2, Subtract2/2
  Add1/1 -> Subtract3/1
  Add3/1 -> Gain/1
  Gain/1 -> Out/1

== system ACDCMG_woPV/Grid Bi-directional Converter 1.2 300 (DC) // 150 V (AC) P_nom 3kW1/Power Measurement (Three-Phase)/Discrete/Phase-B V/Corrected discrete transport delay ==
  In : Inport
  Add1 : Sum
  Add2 : Sum
  Add3 : Sum
  Delay : Delay  DelayLength=ceil(1/F/Ts)-1
  Gain : Gain  Gain=0.5
  Subtract{1..4} (4 alike) : Sum  Inputs=+-
  Unit Delay1 : UnitDelay  SampleTime=Ts  HasFrameUpgradeWarning=on
  Unit Delay2 : UnitDelay  SampleTime=Ts  HasFrameUpgradeWarning=on
  delta : Gain  Gain=(1/F/Ts) - (ceil(1/F/Ts)-1)
  delta' : Gain  Gain=ceil(1/F/Ts) - (1/F/Ts)
  Out : Outport  VectorParamsAs1DForOutWhenUnconnected=off
  wires:
  Gain/1 -> Out/1
  Add3/1 -> Gain/1
  Add1/1 -> Subtract3/1
  Unit Delay2/1 -> Subtract2/2, Add2/2, Subtract3/2
  delta/1 -> Add1/1
  delta'/1 -> Add2/1
  Subtract2/1 -> delta'/1
  Subtract4/1 -> Add3/2
  In/1 -> Subtract1/1, Unit Delay1/1, Subtract4/1, Delay/1
  Unit Delay1/1 -> Add1/2, Subtract1/2
  Delay/1 -> Unit Delay2/1, Subtract2/1
  Subtract3/1 -> Add3/1
  Subtract1/1 -> delta/1
  Add2/1 -> Subtract4/2

== system ACDCMG_woPV/Grid Bi-directional Converter 1.2 300 (DC) // 150 V (AC) P_nom 3kW1/Power Measurement (Three-Phase)/Discrete/Phase-C I/Corrected discrete transport delay ==
  In : Inport
  Add1 : Sum
  Add2 : Sum
  Add3 : Sum
  Delay : Delay  DelayLength=ceil(1/F/Ts)-1
  Gain : Gain  Gain=0.5
  Subtract{1..4} (4 alike) : Sum  Inputs=+-
  Unit Delay1 : UnitDelay  SampleTime=Ts  HasFrameUpgradeWarning=on
  Unit Delay2 : UnitDelay  SampleTime=Ts  HasFrameUpgradeWarning=on
  delta : Gain  Gain=(1/F/Ts) - (ceil(1/F/Ts)-1)
  delta' : Gain  Gain=ceil(1/F/Ts) - (1/F/Ts)
  Out : Outport  VectorParamsAs1DForOutWhenUnconnected=off
  wires:
  Gain/1 -> Out/1
  Add3/1 -> Gain/1
  Add1/1 -> Subtract3/1
  Unit Delay2/1 -> Subtract2/2, Add2/2, Subtract3/2
  delta/1 -> Add1/1
  delta'/1 -> Add2/1
  Subtract2/1 -> delta'/1
  Subtract4/1 -> Add3/2
  In/1 -> Subtract1/1, Unit Delay1/1, Subtract4/1, Delay/1
  Unit Delay1/1 -> Add1/2, Subtract1/2
  Delay/1 -> Unit Delay2/1, Subtract2/1
  Subtract3/1 -> Add3/1
  Subtract1/1 -> delta/1
  Add2/1 -> Subtract4/2

== system ACDCMG_woPV/Grid Bi-directional Converter 1.2 300 (DC) // 150 V (AC) P_nom 3kW1/Power Measurement (Three-Phase)/Discrete/Phase-C V/Corrected discrete transport delay ==
  In : Inport
  Add1 : Sum
  Add2 : Sum
  Add3 : Sum
  Delay : Delay  DelayLength=ceil(1/F/Ts)-1
  Gain : Gain  Gain=0.5
  Subtract{1..4} (4 alike) : Sum  Inputs=+-
  Unit Delay1 : UnitDelay  SampleTime=Ts  HasFrameUpgradeWarning=on
  Unit Delay2 : UnitDelay  SampleTime=Ts  HasFrameUpgradeWarning=on
  delta : Gain  Gain=(1/F/Ts) - (ceil(1/F/Ts)-1)
  delta' : Gain  Gain=ceil(1/F/Ts) - (1/F/Ts)
  Out : Outport  VectorParamsAs1DForOutWhenUnconnected=off
  wires:
  Add2/1 -> Subtract4/2
  Subtract1/1 -> delta/1
  Subtract3/1 -> Add3/1
  Delay/1 -> Subtract2/1, Unit Delay2/1
  Unit Delay1/1 -> Subtract1/2, Add1/2
  In/1 -> Delay/1, Subtract4/1, Unit Delay1/1, Subtract1/1
  Subtract4/1 -> Add3/2
  Subtract2/1 -> delta'/1
  delta'/1 -> Add2/1
  delta/1 -> Add1/1
  Unit Delay2/1 -> Subtract3/2, Add2/2, Subtract2/2
  Add1/1 -> Subtract3/1
  Add3/1 -> Gain/1
  Gain/1 -> Out/1

== system ACDCMG_woPV/Grid Bi-directional Converter 1.2 300 (DC) // 150 V (AC) P_nom 3kW2/Control of Inverter/V//F/UIcontrol/PWM Generator ==
  note: PWM Generator
  note: Pierre Giroux, Gilbert Sybille
      | Power System Laboratory, IREQ
      | Hydro-Quebec
  Signal(s) : Inport  PortDimensions=Signal_PortWidth
  BL4 : Logic  Operator=NOT  Inputs=1
  BL5 : Logic  Operator=NOT  Inputs=1
  Constant : Constant  Value=Internal_Phase
  Constant1 : Constant  Value=Internal
  Data Type Conversion : DataTypeConversion  OutDataTypeStr=double
  Data Type Conversion1 : DataTypeConversion  OutDataTypeStr=boolean
  Data Type Conversion2 : DataTypeConversion  OutDataTypeStr=boolean
  Gain : Gain  Gain=2*pi*Freq  SaturateOnIntegerOverflow=on  OutDataTypeStr=Inherit: Same as input  ParamDataTypeStr=Inherit: Same as input
  Gain2 : Gain  Gain=pi/180  SaturateOnIntegerOverflow=on  OutDataTypeStr=Inherit: Same as input  ParamDataTypeStr=Inherit: Same as input
  Gain3 : Gain  Gain=-1  SaturateOnIntegerOverflow=on  OutDataTypeStr=Inherit: Same as input  ParamDataTypeStr=Inherit: Same as input
  Mux : Mux  Inputs=2
  Mux1 : Mux  Inputs=2
  Mux2 : Mux  Inputs=2
  Product : Product  InputSameDT=on  SaturateOnIntegerOverflow=on  OutDataTypeStr=Inherit: Same as first input
  Relational Operator : RelationalOperator  ZeroCross=off
  Relational Operator1 : RelationalOperator  ZeroCross=off
  Select1A : Selector  InputPortWidth=Select1_PortWidth  IndexOptions=Index vector (dialog)  Indices=Select1_Elements  OutputSizes=1
  Select1B : Selector  InputPortWidth=Select1_PortWidth  IndexOptions=Index vector (dialog)  Indices=Select1_Elements  OutputSizes=1
  Select3 : Selector  InputPortWidth=Select3_PortWidth  IndexOptions=Index vector (dialog)  Indices=Select3_Elements  OutputSizes=1
  Sum : Sum  Inputs=+++  InputSameDT=on  SaturateOnIntegerOverflow=on  OutDataTypeStr=Inherit: Same as first input
  Switch : Switch  Threshold=0.5  SaturateOnIntegerOverflow=off
  Triangle : simulink/Sources/Repeating Sequence  rep_seq_t=[0 1/Fc/4 3/Fc/4 1/Fc]  rep_seq_y=[0 -1 1 0]
  Trigonometric Function : Trigonometry
  m3 : Constant  Value=Phase
  m4 : Constant  Value=mIndex
  t : Clock
  Pulses : Outport
  wires:
  Data Type Conversion2/1 -> Mux1/1, BL5/1
  Relational Operator1/1 -> Data Type Conversion2/1
  Data Type Conversion1/1 -> Mux/1, BL4/1
  Relational Operator/1 -> Data Type Conversion1/1
  Data Type Conversion/1 -> Pulses/1
  Select3/1 -> Data Type Conversion/1
  t/1 -> Gain/1
  Gain/1 -> Sum/1
  Gain2/1 -> Sum/2
  m3/1 -> Gain2/1
  Constant/1 -> Sum/3
  m4/1 -> Product/1
  Sum/1 -> Trigonometric Function/1
  Trigonometric Function/1 -> Product/2
  Signal(s)/1 -> Switch/3
  Constant1/1 -> Switch/2
  Product/1 -> Switch/1
  Gain3/1 -> Relational Operator1/1
  BL4/1 -> Mux/2
  BL5/1 -> Mux1/2
  Mux/1 -> Select1A/1
  Mux1/1 -> Select1B/1
  Select1A/1 -> Mux2/1
  Select1B/1 -> Mux2/2
  Mux2/1 -> Select3/1
  Switch/1 -> Gain3/1, Relational Operator/1
  Triangle/1 -> Relational Operator1/2, Relational Operator/2

== system ACDCMG_woPV/Grid Bi-directional Converter 1.2 300 (DC) // 150 V (AC) P_nom 3kW2/Control of Inverter/V//F/UIcontrol/WL ==
  In1 : Inport
  freq : Inport  Port=2
  L : Inport  Port=3
  2pai : Constant  Value=2*pi
  Product : Product  Inputs=**
  Product1 : Product  Inputs=***
  Out1 : Outport
  wires:
  2pai/1 -> Product/2
  L/1 -> Product1/3
  freq/1 -> Product/1
  Product1/1 -> Out1/1
  Product/1 -> Product1/2
  In1/1 -> Product1/1

== system ACDCMG_woPV/Grid Bi-directional Converter 1.2 300 (DC) // 150 V (AC) P_nom 3kW2/Control of Inverter/V//F/UIcontrol/wC ==
  ed : Inport
  w : Inport  Port=2
  C : Inport  Port=3
  eq : Inport  Port=4
  Product1 : Product  Inputs=3
  Product2 : Product  Inputs=3
  wC ed : Outport
  wC eq : Outport  Port=2
  wires:
  C/1 -> Product1/3, Product2/2
  Product1/1 -> wC ed/1
  w/1 -> Product1/2, Product2/1
  ed/1 -> Product1/1
  eq/1 -> Product2/3
  Product2/1 -> wC eq/1

== system ACDCMG_woPV/Grid Bi-directional Converter 1.2 300 (DC) // 150 V (AC) P_nom 3kW2/Control of Inverter/V//F/UIcontrol/wC1 ==
  id : Inport
  w : Inport  Port=2
  L : Inport  Port=3
  iq : Inport  Port=4
  Product1 : Product  Inputs=***
  Product2 : Product  Inputs=***
  wL id : Outport
  wL iq : Outport  Port=2
  wires:
  L/1 -> Product1/3, Product2/2
  Product1/1 -> wL id/1
  w/1 -> Product1/2, Product2/1
  id/1 -> Product1/1
  iq/1 -> Product2/3
  Product2/1 -> wL iq/1

== system ACDCMG_woPV/Grid Bi-directional Converter 1.2 300 (DC) // 150 V (AC) P_nom 3kW3/Control of Inverter/V//F/UIcontrol/PWM Generator ==
  note: PWM Generator
  note: Pierre Giroux, Gilbert Sybille
      | Power System Laboratory, IREQ
      | Hydro-Quebec
  Signal(s) : Inport  PortDimensions=Signal_PortWidth
  BL4 : Logic  Operator=NOT  Inputs=1
  BL5 : Logic  Operator=NOT  Inputs=1
  Constant : Constant  Value=Internal_Phase
  Constant1 : Constant  Value=Internal
  Data Type Conversion : DataTypeConversion  OutDataTypeStr=double
  Data Type Conversion1 : DataTypeConversion  OutDataTypeStr=boolean
  Data Type Conversion2 : DataTypeConversion  OutDataTypeStr=boolean
  Gain : Gain  Gain=2*pi*Freq  SaturateOnIntegerOverflow=on  OutDataTypeStr=Inherit: Same as input  ParamDataTypeStr=Inherit: Same as input
  Gain2 : Gain  Gain=pi/180  SaturateOnIntegerOverflow=on  OutDataTypeStr=Inherit: Same as input  ParamDataTypeStr=Inherit: Same as input
  Gain3 : Gain  Gain=-1  SaturateOnIntegerOverflow=on  OutDataTypeStr=Inherit: Same as input  ParamDataTypeStr=Inherit: Same as input
  Mux : Mux  Inputs=2
  Mux1 : Mux  Inputs=2
  Mux2 : Mux  Inputs=2
  Product : Product  InputSameDT=on  SaturateOnIntegerOverflow=on  OutDataTypeStr=Inherit: Same as first input
  Relational Operator : RelationalOperator  ZeroCross=off
  Relational Operator1 : RelationalOperator  ZeroCross=off
  Select1A : Selector  InputPortWidth=Select1_PortWidth  IndexOptions=Index vector (dialog)  Indices=Select1_Elements  OutputSizes=1
  Select1B : Selector  InputPortWidth=Select1_PortWidth  IndexOptions=Index vector (dialog)  Indices=Select1_Elements  OutputSizes=1
  Select3 : Selector  InputPortWidth=Select3_PortWidth  IndexOptions=Index vector (dialog)  Indices=Select3_Elements  OutputSizes=1
  Sum : Sum  Inputs=+++  InputSameDT=on  SaturateOnIntegerOverflow=on  OutDataTypeStr=Inherit: Same as first input
  Switch : Switch  Threshold=0.5  SaturateOnIntegerOverflow=off
  Triangle : simulink/Sources/Repeating Sequence  rep_seq_t=[0 1/Fc/4 3/Fc/4 1/Fc]  rep_seq_y=[0 -1 1 0]
  Trigonometric Function : Trigonometry
  m3 : Constant  Value=Phase
  m4 : Constant  Value=mIndex
  t : Clock
  Pulses : Outport
  wires:
  Data Type Conversion2/1 -> Mux1/1, BL5/1
  Relational Operator1/1 -> Data Type Conversion2/1
  Data Type Conversion1/1 -> Mux/1, BL4/1
  Relational Operator/1 -> Data Type Conversion1/1
  Data Type Conversion/1 -> Pulses/1
  Select3/1 -> Data Type Conversion/1
  t/1 -> Gain/1
  Gain/1 -> Sum/1
  Gain2/1 -> Sum/2
  m3/1 -> Gain2/1
  Constant/1 -> Sum/3
  m4/1 -> Product/1
  Sum/1 -> Trigonometric Function/1
  Trigonometric Function/1 -> Product/2
  Signal(s)/1 -> Switch/3
  Constant1/1 -> Switch/2
  Product/1 -> Switch/1
  Gain3/1 -> Relational Operator1/1
  BL4/1 -> Mux/2
  BL5/1 -> Mux1/2
  Mux/1 -> Select1A/1
  Mux1/1 -> Select1B/1
  Select1A/1 -> Mux2/1
  Select1B/1 -> Mux2/2
  Mux2/1 -> Select3/1
  Switch/1 -> Gain3/1, Relational Operator/1
  Triangle/1 -> Relational Operator1/2, Relational Operator/2

== system ACDCMG_woPV/Grid Bi-directional Converter 1.2 300 (DC) // 150 V (AC) P_nom 3kW3/Control of Inverter/V//F/UIcontrol/WL ==
  In1 : Inport
  freq : Inport  Port=2
  L : Inport  Port=3
  2pai : Constant  Value=2*pi
  Product : Product  Inputs=**
  Product1 : Product  Inputs=***
  Out1 : Outport
  wires:
  2pai/1 -> Product/2
  L/1 -> Product1/3
  freq/1 -> Product/1
  Product1/1 -> Out1/1
  Product/1 -> Product1/2
  In1/1 -> Product1/1

== system ACDCMG_woPV/Grid Bi-directional Converter 1.2 300 (DC) // 150 V (AC) P_nom 3kW3/Control of Inverter/V//F/UIcontrol/wC ==
  ed : Inport
  w : Inport  Port=2
  C : Inport  Port=3
  eq : Inport  Port=4
  Product1 : Product  Inputs=3
  Product2 : Product  Inputs=3
  wC ed : Outport
  wC eq : Outport  Port=2
  wires:
  C/1 -> Product1/3, Product2/2
  Product1/1 -> wC ed/1
  w/1 -> Product1/2, Product2/1
  ed/1 -> Product1/1
  eq/1 -> Product2/3
  Product2/1 -> wC eq/1

== system ACDCMG_woPV/Grid Bi-directional Converter 1.2 300 (DC) // 150 V (AC) P_nom 3kW3/Control of Inverter/V//F/UIcontrol/wC1 ==
  id : Inport
  w : Inport  Port=2
  L : Inport  Port=3
  iq : Inport  Port=4
  Product1 : Product  Inputs=***
  Product2 : Product  Inputs=***
  wL id : Outport
  wL iq : Outport  Port=2
  wires:
  L/1 -> Product1/3, Product2/2
  Product1/1 -> wL id/1
  w/1 -> Product1/2, Product2/1
  id/1 -> Product1/1
  iq/1 -> Product2/3
  Product2/1 -> wL iq/1

== system ACDCMG_woPV/Inverter 300 (DC) // 150 V (AC) P_nom 3kW4/Control of Inverter/V//F/UIcontrol/PWM Generator ==
  note: PWM Generator
  note: Pierre Giroux, Gilbert Sybille
      | Power System Laboratory, IREQ
      | Hydro-Quebec
  Signal(s) : Inport  PortDimensions=Signal_PortWidth
  BL4 : Logic  Operator=NOT  Inputs=1
  BL5 : Logic  Operator=NOT  Inputs=1
  Constant : Constant  Value=Internal_Phase
  Constant1 : Constant  Value=Internal
  Data Type Conversion : DataTypeConversion  OutDataTypeStr=double
  Data Type Conversion1 : DataTypeConversion  OutDataTypeStr=boolean
  Data Type Conversion2 : DataTypeConversion  OutDataTypeStr=boolean
  Gain : Gain  Gain=2*pi*Freq  SaturateOnIntegerOverflow=on  OutDataTypeStr=Inherit: Same as input  ParamDataTypeStr=Inherit: Same as input
  Gain2 : Gain  Gain=pi/180  SaturateOnIntegerOverflow=on  OutDataTypeStr=Inherit: Same as input  ParamDataTypeStr=Inherit: Same as input
  Gain3 : Gain  Gain=-1  SaturateOnIntegerOverflow=on  OutDataTypeStr=Inherit: Same as input  ParamDataTypeStr=Inherit: Same as input
  Mux : Mux  Inputs=2
  Mux1 : Mux  Inputs=2
  Mux2 : Mux  Inputs=2
  Product : Product  InputSameDT=on  SaturateOnIntegerOverflow=on  OutDataTypeStr=Inherit: Same as first input
  Relational Operator : RelationalOperator  ZeroCross=off
  Relational Operator1 : RelationalOperator  ZeroCross=off
  Select1A : Selector  InputPortWidth=Select1_PortWidth  IndexOptions=Index vector (dialog)  Indices=Select1_Elements  OutputSizes=1
  Select1B : Selector  InputPortWidth=Select1_PortWidth  IndexOptions=Index vector (dialog)  Indices=Select1_Elements  OutputSizes=1
  Select3 : Selector  InputPortWidth=Select3_PortWidth  IndexOptions=Index vector (dialog)  Indices=Select3_Elements  OutputSizes=1
  Sum : Sum  Inputs=+++  InputSameDT=on  SaturateOnIntegerOverflow=on  OutDataTypeStr=Inherit: Same as first input
  Switch : Switch  Threshold=0.5  SaturateOnIntegerOverflow=off
  Triangle : simulink/Sources/Repeating Sequence  rep_seq_t=[0 1/Fc/4 3/Fc/4 1/Fc]  rep_seq_y=[0 -1 1 0]
  Trigonometric Function : Trigonometry
  m3 : Constant  Value=Phase
  m4 : Constant  Value=mIndex
  t : Clock
  Pulses : Outport
  wires:
  Data Type Conversion2/1 -> Mux1/1, BL5/1
  Relational Operator1/1 -> Data Type Conversion2/1
  Data Type Conversion1/1 -> Mux/1, BL4/1
  Relational Operator/1 -> Data Type Conversion1/1
  Data Type Conversion/1 -> Pulses/1
  Select3/1 -> Data Type Conversion/1
  t/1 -> Gain/1
  Gain/1 -> Sum/1
  Gain2/1 -> Sum/2
  m3/1 -> Gain2/1
  Constant/1 -> Sum/3
  m4/1 -> Product/1
  Sum/1 -> Trigonometric Function/1
  Trigonometric Function/1 -> Product/2
  Signal(s)/1 -> Switch/3
  Constant1/1 -> Switch/2
  Product/1 -> Switch/1
  Gain3/1 -> Relational Operator1/1
  BL4/1 -> Mux/2
  BL5/1 -> Mux1/2
  Mux/1 -> Select1A/1
  Mux1/1 -> Select1B/1
  Select1A/1 -> Mux2/1
  Select1B/1 -> Mux2/2
  Mux2/1 -> Select3/1
  Switch/1 -> Gain3/1, Relational Operator/1
  Triangle/1 -> Relational Operator1/2, Relational Operator/2

== system ACDCMG_woPV/Inverter 300 (DC) // 150 V (AC) P_nom 3kW4/Control of Inverter/V//F/UIcontrol/WL ==
  In1 : Inport
  freq : Inport  Port=2
  L : Inport  Port=3
  2pai : Constant  Value=2*pi
  Product : Product  Inputs=**
  Product1 : Product  Inputs=***
  Out1 : Outport
  wires:
  2pai/1 -> Product/2
  L/1 -> Product1/3
  freq/1 -> Product/1
  Product1/1 -> Out1/1
  Product/1 -> Product1/2
  In1/1 -> Product1/1

== system ACDCMG_woPV/Inverter 300 (DC) // 150 V (AC) P_nom 3kW4/Control of Inverter/V//F/UIcontrol/wC ==
  ed : Inport
  w : Inport  Port=2
  C : Inport  Port=3
  eq : Inport  Port=4
  Product1 : Product  Inputs=3
  Product2 : Product  Inputs=3
  wC ed : Outport
  wC eq : Outport  Port=2
  wires:
  C/1 -> Product1/3, Product2/2
  Product1/1 -> wC ed/1
  w/1 -> Product1/2, Product2/1
  ed/1 -> Product1/1
  eq/1 -> Product2/3
  Product2/1 -> wC eq/1

== system ACDCMG_woPV/Inverter 300 (DC) // 150 V (AC) P_nom 3kW4/Control of Inverter/V//F/UIcontrol/wC1 ==
  id : Inport
  w : Inport  Port=2
  L : Inport  Port=3
  iq : Inport  Port=4
  Product1 : Product  Inputs=***
  Product2 : Product  Inputs=***
  wL id : Outport
  wL iq : Outport  Port=2
  wires:
  L/1 -> Product1/3, Product2/2
  Product1/1 -> wL id/1
  w/1 -> Product1/2, Product2/1
  id/1 -> Product1/1
  iq/1 -> Product2/3
  Product2/1 -> wL iq/1
